simulink subsystem "PWM_BOX"  (R2020b)
settings: Solver=VariableStepAuto  StartTime=0.0  StopTime=10.0  RelTol=1e-3
settings Model: Creator=lee884  LastModifiedBy=lee884

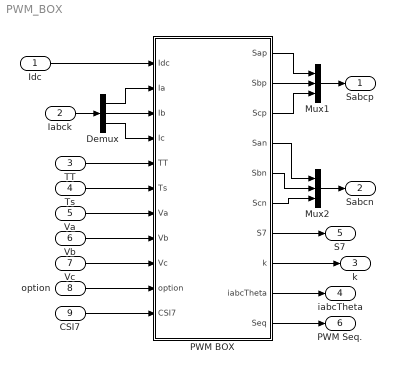
== system PWM_BOX ==
  Idc : Inport
  Iabck : Inport  Port=2
  TT : Inport  Port=3
  Ts : Inport  Port=4
  Va : Inport  Port=5
  Vb : Inport  Port=6
  Vc : Inport  Port=7
  option : Inport  Port=8
  CSI7 : Inport  Port=9
  Demux : Demux  Outputs=3
  Mux1 : Mux  Inputs=3
  Mux2 : Mux  Inputs=3
  PWM BOX : MATLAB Function  TreatAsAtomicUnit=on
  Sabcp : Outport
  Sabcn : Outport  Port=2
  k : Outport  Port=3
  iabcTheta : Outport  Port=4
  S7 : Outport  Port=5
  PWM Seq. : Outport  Port=6
  wires:
  Demux/2 -> PWM BOX/3(Ib)
  PWM BOX/9(iabcTheta) -> iabcTheta/1
  PWM BOX/2(Sbp) -> Mux1/2
  PWM BOX/6(Scn) -> Mux2/3
  PWM BOX/4(San) -> Mux2/1
  Demux/1 -> PWM BOX/2(Ia)
  PWM BOX/5(Sbn) -> Mux2/2
  PWM BOX/3(Scp) -> Mux1/3
  PWM BOX/8(k) -> k/1
  Demux/3 -> PWM BOX/4(Ic)
  TT/1 -> PWM BOX/5(TT)
  PWM BOX/1(Sap) -> Mux1/1
  Mux1/1 -> Sabcp/1
  Ts/1 -> PWM BOX/6(Ts)
  Mux2/1 -> Sabcn/1
  Idc/1 -> PWM BOX/1(Idc)
  Iabck/1 -> Demux/1
  option/1 -> PWM BOX/10(option)
  CSI7/1 -> PWM BOX/11(CSI7)
  PWM BOX/7(S7) -> S7/1
  Va/1 -> PWM BOX/7(Va)
  Vb/1 -> PWM BOX/8(Vb)
  Vc/1 -> PWM BOX/9(Vc)
  PWM BOX/10(Seq) -> PWM Seq./1

== matlab function PWM_BOX/PWM BOX ==
  data: Idc input; Sap output; Sbp output; Scp output; Ia input; Ib input; Ic input; TT input; San output; Ts input; Va input; Vb input; Vc input; Sbn output; Scn output; S7 output; k output; iabcTheta output; option input; CSI7 input; Seq output
function [Sap, Sbp, Scp, San, Sbn, Scn, S7, k,iabcTheta, Seq] = CSI_SVPWM(Idc, Ia, Ib, Ic, TT, Ts, Va, Vb, Vc, option, CSI7)

% S0 = [];
% S1 = [];
% S2 = [];
%% Current space vector
iabc = 2/3 * ( Ia + Ib*exp(1j*2*pi/3) + Ic*exp(1j*4*pi/3) );

%% Sector indentification
iabcTheta = angle (iabc)*180/pi;          % [deg] -180 ~ 180
Seq = 0;
%% CSI switching states
Sab = [1 0 0, 0 1 0];
Sac = [1 0 0, 0 0 1];
Sbc = [0 1 0, 0 0 1];
Sba = [0 1 0, 1 0 0];
Sca = [0 0 1, 1 0 0];
Scb = [0 0 1, 0 1 0];
Saa = [1 0 0, 1 0 0];
Sbb = [0 1 0, 0 1 0];
Scc = [0 0 1, 0 0 1];

%% Sector Identification
k = sector_cal(iabcTheta);

%% Calculate T1, T2, T0 and new T1, T2, T0
[T1, T2, T0] = dwell_time_cal(iabc,iabcTheta,k);
[T1New, T2New] = new_dwell_time_cal(T1, T2, T0);

%% PWM Mapping S0 S1 S2 to switching states
switch option
    case 0
        [Sap, Sbp, Scp, San, Sbn, Scn] = CSM1A(k,TT,Ts,Saa,Sbb,Scc,Sab,Sac,Sbc,Sba,Sca,Scb);
    case 1
        [Sap, Sbp, Scp, San, Sbn, Scn] = DL_CSM1A(k,TT,Ts,Saa,Sbb,Scc,Sab,Sac,Sbc,Sba,Sca,Scb);
    case 2
        [Sap, Sbp, Scp, San, Sbn, Scn] = CSM2A(k,TT,Ts,Saa,Sbb,Scc,Sab,Sac,Sbc,Sba,Sca,Scb);
    case 3
        [Sap, Sbp, Scp, San, Sbn, Scn] = DL_CSM2A(k,TT,Ts,Saa,Sbb,Scc,Sab,Sac,Sbc,Sba,Sca,Scb);
    case 4
        [Sap, Sbp, Scp, San, Sbn, Scn] = CSM3A(k,TT,Ts,Saa,Sbb,Scc,Sab,Sac,Sbc,Sba,Sca,Scb);
        %[Sap, Sbp, Scp, San, Sbn, Scn, S7] = CSM3A_CSI7_with_overlap(k,TT,Ts,Saa,Sbb,Scc,Sab,Sac,Sbc,Sba,Sca,Scb);
    case 5
        [Sap, Sbp, Scp, San, Sbn, Scn] = CSM3A_BoostMinus60deg(k,TT,Ts,Saa,Sbb,Scc,Sab,Sac,Sbc,Sba,Sca,Scb);
    case 6 
        [Sap, Sbp, Scp, San, Sbn, Scn] = AVM(k,TT,Ts,Saa,Sbb,Scc,Sab,Sac,Sbc,Sba,Sca,Scb,Va,Vb,Vc);
    case 7
        [Sap, Sbp, Scp, San, Sbn, Scn] = CSM1B(k,TT,Ts,Saa,Sbb,Scc,Sab,Sac,Sbc,Sba,Sca,Scb);
    case 8
        [Sap, Sbp, Scp, San, Sbn, Scn] = AVM3(k,TT,Ts,Saa,Sbb,Scc,Sab,Sac,Sbc,Sba,Sca,Scb,Va,Vb,Vc);
    otherwise
        [Sap, Sbp, Scp, San, Sbn, Scn, Seq] = ASVM(k,TT,Ts,Saa,Sbb,Scc,Sab,Sac,Sbc,Sba,Sca,Scb,Va,Vb,Vc);        
        
end

%% for CSI7 case, this is the correct modulation of S7 without overlap
if(CSI7 == 1)
    [Sap, Sbp, Scp, San, Sbn, Scn, S7] = S7_modulation(Sap, Sbp, Scp, San, Sbn, Scn);
else
    S7 = 0;
end

% if(option == 4)
%     [Sap, Sbp, Scp, San, Sbn, Scn, S7] = CSM3A_CSI7_with_overlap(k,TT,Ts,Saa,Sbb,Scc,Sab,Sac,Sbc,Sba,Sca,Scb);
% end

%% Define nested functions

    %% Dwell time calculation
    function [T1, T2, T0] = dwell_time_cal(iabc, iabcTheta, k)        
        iabcThetaSector = iabcTheta*pi/180 - (k-1)*pi/3;       % [rad]
        T1 = abs(iabc)/Idc * sin(pi/6-iabcThetaSector) * Ts; 
        T2= abs(iabc)/Idc * sin(pi/6+iabcThetaSector) * Ts; 
        T0 = Ts-T1-T2;
    end

    %% Dwell time calculation for wrong CSI7 or PWAM
    function [T1New, T2New] = new_dwell_time_cal(T1, T2, T0)
        T1New = T1/(T1+T2)*Ts;
        T2New = T2/(T1+T2)*Ts;
    end

    %% Sector number k cacluation
    function k = sector_cal(iabcTheta)
        if iabcTheta > -30 && iabcTheta <= 0; k=1; 
        elseif iabcTheta > 0 && iabcTheta <= 30; k=1;  
    
        % Sector 2
        elseif iabcTheta > 30 && iabcTheta <= 90; k=2; 
    
        % Sector 3
        elseif iabcTheta > 90 && iabcTheta <= 150; k=3; 
    
        % Sector 4
        elseif iabcTheta > 150 && iabcTheta <= 180; k=4; 
        elseif iabcTheta > -180 && iabcTheta <= -150; k=4; 
    
        % Sector 5
        elseif iabcTheta > -150 && iabcTheta <= -90; k=5; 
    
        % Sector 6
        elseif iabcTheta > -90 && iabcTheta <= -30; k=6; 
    
        % Else- Error
        else k = 10; 
        end        
    end



%%%%%%%%%%%%%%%%%%%%%%%%%%%%%%%%%%%%%%%%%%%%%%%%% PWM logics
%%%%%%%%%%%%%%%%%%%%%%%%%%%%%%%%%%%%%%%%%%%%%%%%% %%%%%%%%%%%%%%%%%%%%%%%%%%%%%%%%%%%%%%%
%% CSM1A: IZ-IA-IB-IA-IZ
% CSM1A
    function [Sap, Sbp, Scp, San, Sbn, Scn] = CSM1A(k,TT,Ts,Saa,Sbb,Scc,Sab,Sac,Sbc,Sba,Sca,Scb)
        
        switch k
            case 1
                S0 = Saa; S1 = Sab; S2 = Sac;
            case 2
                S0 = Scc; S1 = Sac; S2 = Sbc;
            case 3
                S0 = Sbb; S1 = Sbc; S2 = Sba;
            case 4
                S0 = Saa; S1 = Sba; S2 = Sca;
            case 5
                S0 = Scc; S1 = Sca; S2 = Scb;
            case 6
                S0 = Sbb; S1 = Scb; S2 = Sab;
            otherwise
                S0 = Saa; S1 = Sab; S2 = Sac;
        end
        
        
        % initialize switching functions
        Sap = 1; Sbp = 1; Scp = 1;
        San = 1; Sbn = 1; Scn = 1;
        
        % PWM sequence: IZ-IA-IB-IA-IZ
        if TT>=0 && TT<T0/2
            % aa or bb or cc, CSI zero state
            Sap = S0(1);    Sbp = S0(2);    Scp = S0(3);
            San = S0(4);    Sbn = S0(5);    Scn = S0(6);

        elseif TT>=T0/2 && TT<T0/2 + T1/2
            % T1 state
            Sap = S1(1);    Sbp = S1(2);    Scp = S1(3);
            San = S1(4);    Sbn = S1(5);    Scn = S1(6);    

        elseif TT>=T0/2 + T1/2 && TT<=T0/2 + T1/2 +T2 
            % T2 state
            Sap = S2(1);    Sbp = S2(2);    Scp = S2(3);
            San = S2(4);    Sbn = S2(5);    Scn = S2(6);
    
        elseif TT>=T0/2 + T1/2 +T2 && TT<T0/2 + T1 +T2
            % T1 state
            Sap = S1(1);    Sbp = S1(2);    Scp = S1(3);
            San = S1(4);    Sbn = S1(5);    Scn = S1(6);

        elseif TT>=T0/2 + T1 +T2 && TT<Ts
            % aa or bb or cc, CSI zero state
            Sap = S0(1);    Sbp = S0(2);    Scp = S0(3);
            San = S0(4);    Sbn = S0(5);    Scn = S0(6);
        end        
    end

%% CSM1B: IZ-IB-IA-IB-IZ
% CSM1B
    function [Sap, Sbp, Scp, San, Sbn, Scn] = CSM1B(k,TT,Ts,Saa,Sbb,Scc,Sab,Sac,Sbc,Sba,Sca,Scb)
        
        switch k
            case 1
                S0 = Saa; S1 = Sab; S2 = Sac;
            case 2
                S0 = Scc; S1 = Sac; S2 = Sbc;
            case 3
                S0 = Sbb; S1 = Sbc; S2 = Sba;
            case 4
                S0 = Saa; S1 = Sba; S2 = Sca;
            case 5
                S0 = Scc; S1 = Sca; S2 = Scb;
            case 6
                S0 = Sbb; S1 = Scb; S2 = Sab;
            otherwise
                S0 = Saa; S1 = Sab; S2 = Sac;
        end
        
        
        % initialize switching functions
        Sap = 1; Sbp = 1; Scp = 1;
        San = 1; Sbn = 1; Scn = 1;
        
        % PWM sequence: IZ-IB-IA-IB-IZ
        if TT>=0 && TT<T0/2
            % aa or bb or cc, CSI zero state
            Sap = S0(1);    Sbp = S0(2);    Scp = S0(3);
            San = S0(4);    Sbn = S0(5);    Scn = S0(6);

        elseif TT>=T0/2 && TT<T0/2 + T2/2
            % T1 state
            Sap = S2(1);    Sbp = S2(2);    Scp = S2(3);
            San = S2(4);    Sbn = S2(5);    Scn = S2(6);    

        elseif TT>=T0/2 + T2/2 && TT<=T0/2 + T2/2 +T1 
            % T2 state
            Sap = S1(1);    Sbp = S1(2);    Scp = S1(3);
            San = S1(4);    Sbn = S1(5);    Scn = S1(6);
    
        elseif TT>=T0/2 + T2/2 +T1 && TT<T0/2 + T2 +T1
            % T1 state
            Sap = S2(1);    Sbp = S2(2);    Scp = S2(3);
            San = S2(4);    Sbn = S2(5);    Scn = S2(6);

        elseif TT>=T0/2 + T2 + T1 && TT<Ts
            % aa or bb or cc, CSI zero state
            Sap = S0(1);    Sbp = S0(2);    Scp = S0(3);
            San = S0(4);    Sbn = S0(5);    Scn = S0(6);
        end        
    end

%% DL-CSM1A: IZ-IA-IB-IA-IZ
% DL-CSM1A
    function [Sap, Sbp, Scp, San, Sbn, Scn] = DL_CSM1A(k,TT,Ts,Saa,Sbb,Scc,Sab,Sac,Sbc,Sba,Sca,Scb)
        switch k
            case 1
                S0 = Sbb; S1 = Sab; S2 = Sac;
            case 2
                S0 = Saa; S1 = Sac; S2 = Sbc;
            case 3
                S0 = Scc; S1 = Sbc; S2 = Sba;
            case 4
                S0 = Sbb; S1 = Sba; S2 = Sca;
            case 5
                S0 = Saa; S1 = Sca; S2 = Scb;
            case 6
                S0 = Scc; S1 = Scb; S2 = Sab;
            otherwise
                S0 = Saa; S1 = Sab; S2 = Sac;
        end

        % initialize switching functions
        Sap = 1; Sbp = 1; Scp = 1;
        San = 1; Sbn = 1; Scn = 1;        
        
        % PWM sequence: IZ-IA-IB-IA-IZ
        if TT>=0 && TT<T0/2
            % aa or bb or cc, CSI zero state
            Sap = S0(1);    Sbp = S0(2);    Scp = S0(3);
            San = S0(4);    Sbn = S0(5);    Scn = S0(6);

        elseif TT>=T0/2 && TT<T0/2 + T1/2
            % T1 state
            Sap = S1(1);    Sbp = S1(2);    Scp = S1(3);
            San = S1(4);    Sbn = S1(5);    Scn = S1(6);    

        elseif TT>=T0/2 + T1/2 && TT<=T0/2 + T1/2 +T2 
            % T2 state
            Sap = S2(1);    Sbp = S2(2);    Scp = S2(3);
            San = S2(4);    Sbn = S2(5);    Scn = S2(6);
    
        elseif TT>=T0/2 + T1/2 +T2 && TT<T0/2 + T1 +T2
            % T1 state
            Sap = S1(1);    Sbp = S1(2);    Scp = S1(3);
            San = S1(4);    Sbn = S1(5);    Scn = S1(6);

        elseif TT>=T0/2 + T1 +T2 && TT<Ts
            % aa or bb or cc, CSI zero state
            Sap = S0(1);    Sbp = S0(2);    Scp = S0(3);
            San = S0(4);    Sbn = S0(5);    Scn = S0(6);
        end  
    end

%% CSM2A: IA-IB-IZ-IB-IA
% CSM1A
    function [Sap, Sbp, Scp, San, Sbn, Scn] = CSM2A(k,TT,Ts,Saa,Sbb,Scc,Sab,Sac,Sbc,Sba,Sca,Scb)
        

        switch k
            case 1
                S0 = Saa; S1 = Sab; S2 = Sac;
            case 2
                S0 = Scc; S1 = Sac; S2 = Sbc;
            case 3
                S0 = Sbb; S1 = Sbc; S2 = Sba;
            case 4
                S0 = Saa; S1 = Sba; S2 = Sca;
            case 5
                S0 = Scc; S1 = Sca; S2 = Scb;
            case 6
                S0 = Sbb; S1 = Scb; S2 = Sab;
            otherwise
                S0 = Saa; S1 = Sab; S2 = Sac;
        end
        
        
        % initialize switching functions
        Sap = 1; Sbp = 1; Scp = 1;
        San = 1; Sbn = 1; Scn = 1;
        
        % PWM sequence: IA-IB-IZ-IB-IA
        if TT>=0 && TT<T1/2
            % aa or bb or cc, CSI zero state
            Sap = S1(1);    Sbp = S1(2);    Scp = S1(3);
            San = S1(4);    Sbn = S1(5);    Scn = S1(6);

        elseif TT>=T1/2 && TT<T1/2 + T2/2
            % T1 state
            Sap = S2(1);    Sbp = S2(2);    Scp = S2(3);
            San = S2(4);    Sbn = S2(5);    Scn = S2(6);    

        elseif TT>=T1/2 + T2/2 && TT<=T1/2 + T2/2 + T0 
            % T2 state
            Sap = S0(1);    Sbp = S0(2);    Scp = S0(3);
            San = S0(4);    Sbn = S0(5);    Scn = S0(6);
    
        elseif TT>=T1/2 + T2/2 + T0 && TT<T1/2 + T2 +T0
            % T1 state
            Sap = S2(1);    Sbp = S2(2);    Scp = S2(3);
            San = S2(4);    Sbn = S2(5);    Scn = S2(6);

        elseif TT>=T1/2 + T2 +T0 && TT<Ts
            % aa or bb or cc, CSI zero state
            Sap = S1(1);    Sbp = S1(2);    Scp = S1(3);
            San = S1(4);    Sbn = S1(5);    Scn = S1(6);
        end        
    end

%% DL-CSM2A: IA-IB-IZ-IB-IA
% DL-CSM2A
    function [Sap, Sbp, Scp, San, Sbn, Scn] = DL_CSM2A(k,TT,Ts,Saa,Sbb,Scc,Sab,Sac,Sbc,Sba,Sca,Scb)
        switch k
            case 1
                S0 = Scc; S1 = Sab; S2 = Sac;
            case 2
                S0 = Sbb; S1 = Sac; S2 = Sbc;
            case 3
                S0 = Saa; S1 = Sbc; S2 = Sba;
            case 4
                S0 = Scc; S1 = Sba; S2 = Sca;
            case 5
                S0 = Sbb; S1 = Sca; S2 = Scb;
            case 6
                S0 = Saa; S1 = Scb; S2 = Sab;
            otherwise
                S0 = Saa; S1 = Sab; S2 = Sac;
        end

        % initialize switching functions
        Sap = 1; Sbp = 1; Scp = 1;
        San = 1; Sbn = 1; Scn = 1;        
        
        % PWM sequence: IA-IB-IZ-IB-IA
        if TT>=0 && TT<T1/2
            % aa or bb or cc, CSI zero state
            Sap = S1(1);    Sbp = S1(2);    Scp = S1(3);
            San = S1(4);    Sbn = S1(5);    Scn = S1(6);

        elseif TT>=T1/2 && TT<T1/2 + T2/2
            % T1 state
            Sap = S2(1);    Sbp = S2(2);    Scp = S2(3);
            San = S2(4);    Sbn = S2(5);    Scn = S2(6);    

        elseif TT>=T1/2 + T2/2 && TT<=T1/2 + T2/2 +T0 
            % T2 state
            Sap = S0(1);    Sbp = S0(2);    Scp = S0(3);
            San = S0(4);    Sbn = S0(5);    Scn = S0(6);
    
        elseif TT>=T1/2 + T2/2 +T0 && TT<T1/2 + T2 +T0
            % T1 state
            Sap = S2(1);    Sbp = S2(2);    Scp = S2(3);
            San = S2(4);    Sbn = S2(5);    Scn = S2(6);

        elseif TT>=T1/2 + T2 +T0 && TT<Ts
            % aa or bb or cc, CSI zero state
            Sap = S1(1);    Sbp = S1(2);    Scp = S1(3);
            San = S1(4);    Sbn = S1(5);    Scn = S1(6);
        end  
    end

%% CSI7 or PWAM: IZ-IA-IB-IA-IZ
% Wrong CSI7 modulation
    function [Sap, Sbp, Scp, San, Sbn, Scn, S7] = CSM3A_CSI7_with_overlap(k,TT,Ts,Saa,Sbb,Scc,Sab,Sac,Sbc,Sba,Sca,Scb)
        
        switch k
            case 1
                S0 = Saa; S1 = Sab; S2 = Sac;
            case 2
                S0 = Scc; S1 = Sac; S2 = Sbc;
            case 3
                S0 = Sbb; S1 = Sbc; S2 = Sba;
            case 4
                S0 = Saa; S1 = Sba; S2 = Sca;
            case 5
                S0 = Scc; S1 = Sca; S2 = Scb;
            case 6
                S0 = Sbb; S1 = Scb; S2 = Sab;
            otherwise
                S0 = Saa; S1 = Sab; S2 = Sac;
        end

        % initialize switching functions
        Sap = 1; Sbp = 1; Scp = 1;
        San = 1; Sbn = 1; Scn = 1; 
        S7 = 0;

        % PWM sequence for CSI switch : IZ-IA-IB-IA-IZ
        if TT>=0 && TT<T1New/2
            % aa or bb or cc, CSI zero state
            Sap = S1(1);    Sbp = S1(2);    Scp = S1(3);
            San = S1(4);    Sbn = S1(5);    Scn = S1(6);

        elseif TT>=T1New/2 && TT<T1New/2 + T2New
            % T1 state
            Sap = S2(1);    Sbp = S2(2);    Scp = S2(3);
            San = S2(4);    Sbn = S2(5);    Scn = S2(6);

        elseif TT>=T1New/2 + T2New && TT<Ts 
            % T2 state
            Sap = S1(1);    Sbp = S1(2);    Scp = S1(3);
            San = S1(4);    Sbn = S1(5);    Scn = S1(6);
        end           
        
        
        % PWM sequence for S7 : IZ-IA-IB-IA-IZ
        if TT>=0 && TT<T1/2
            % T1 state
            S7 = 0;

        elseif TT>=T1/2 && TT<T1/2 + T0/2
            % aa or bb or cc, CSI zero state
            S7 = 1;

        elseif TT>=T1/2 + T0/2 && TT< T1/2 + T0/2 +T2 
            % T2 state
            S7 = 0;
    
        elseif TT>=T1/2 + T0/2 +T2 && TT<T1/2 + T0 +T2
            % aa or bb or cc, CSI zero state
            S7 = 1;

        elseif TT>=T1/2 + T0 +T2 && TT<Ts
            % T1 state  
            S7 = 0;
        end        
    end

%% CSM3A IA-IZ-IB-IZ-IA
% CSM3
    function [Sap, Sbp, Scp, San, Sbn, Scn] = CSM3A(k,TT,Ts,Saa,Sbb,Scc,Sab,Sac,Sbc,Sba,Sca,Scb)

        switch k
            case 1
                S0 = Saa; S1 = Sab; S2 = Sac;
            case 2
                S0 = Scc; S1 = Sac; S2 = Sbc;
            case 3
                S0 = Sbb; S1 = Sbc; S2 = Sba;
            case 4
                S0 = Saa; S1 = Sba; S2 = Sca;
            case 5
                S0 = Scc; S1 = Sca; S2 = Scb;
            case 6
                S0 = Sbb; S1 = Scb; S2 = Sab;
            otherwise
                S0 = Saa; S1 = Sab; S2 = Sac;
        end
        
        
        % initialize switching functions
        Sap = 1; Sbp = 1; Scp = 1;
        San = 1; Sbn = 1; Scn = 1;
        
        % PWM sequence: IA-IZ-IB-IZ-IA
        if TT>=0 && TT<T1/2
            % T1
            Sap = S1(1);    Sbp = S1(2);    Scp = S1(3);
            San = S1(4);    Sbn = S1(5);    Scn = S1(6);

        elseif TT>=T1/2 && TT<T1/2 + T0/2
            % T0
            Sap = S0(1);    Sbp = S0(2);    Scp = S0(3);
            San = S0(4);    Sbn = S0(5);    Scn = S0(6);    

        elseif TT>=T1/2 + T2/2 && TT<=T1/2 + T0/2 + T2 
            % T2
            Sap = S2(1);    Sbp = S2(2);    Scp = S2(3);
            San = S2(4);    Sbn = S2(5);    Scn = S2(6);
    
        elseif TT>=T1/2 + T0/2 + T2 && TT<T1/2 + T2 +T0
            % T0
            Sap = S0(1);    Sbp = S0(2);    Scp = S0(3);
            San = S0(4);    Sbn = S0(5);    Scn = S0(6);

        elseif TT>=T1/2 + T2 +T0 && TT<Ts
            % T1
            Sap = S1(1);    Sbp = S1(2);    Scp = S1(3);
            San = S1(4);    Sbn = S1(5);    Scn = S1(6);
        end        
    end

%% S7 modulation with direct replacment of zero vectors
    function [Sap, Sbp, Scp, San, Sbn, Scn, S7] = S7_modulation(Sap, Sbp, Scp, San, Sbn, Scn)
         S7 = 0;
         if(Sap == 1 && San ==1)
             S7 = 1;
             Sap = 0; San = 0;
         end
         
         if(Sbp == 1 && Sbn ==1)
             S7 = 1;
             Sbp = 0; Sbn = 0;
         end
         
         if(Scp == 1 && Scn ==1)
             S7 = 1;
             Scp = 0; Scn = 0;
         end
         
    end

%% boost operation modulation CSM3A IA-IZ-IB-IZ-IA with negative
    function [Sap, Sbp, Scp, San, Sbn, Scn] = CSM3A_BoostMinus60deg(k,TT,Ts,Saa,Sbb,Scc,Sab,Sac,Sbc,Sba,Sca,Scb)
        
        switch k
            case 1
                S0 = Saa; S1 = Sab; S2 = Sbc;
            case 2
                S0 = Scc; S1 = Sac; S2 = Sba;
            case 3
                S0 = Sbb; S1 = Sbc; S2 = Sca;
            case 4
                S0 = Saa; S1 = Sba; S2 = Scb;
            case 5
                S0 = Scc; S1 = Sca; S2 = Sab;
            case 6
                S0 = Sbb; S1 = Scb; S2 = Sac;
            otherwise
                S0 = Saa; S1 = Sab; S2 = Sac;
        end

        % initialize switching functions
        Sap = 1; Sbp = 1; Scp = 1;
        San = 1; Sbn = 1; Scn = 1; 
        S7 = 0;
        
        % For 60 deg T1 becomes T1 + T2 and T2 becomes T2
        T1new = T1 + T2;
        T2new = T2;
        T0new = Ts - T1new - T2new;
        
        % PWM sequence for CSI switch : IA-IZ-IB-IZ-IA
        if TT>=0 && TT<T1new/2
            % T1 state
            Sap = S1(1);    Sbp = S1(2);    Scp = S1(3);
            San = S1(4);    Sbn = S1(5);    Scn = S1(6);

        elseif TT>=T1new/2 && TT<T1new/2 + T0new/2
            % T0 state
            Sap = S0(1);    Sbp = S0(2);    Scp = S0(3);
            San = S0(4);    Sbn = S0(5);    Scn = S0(6);

        elseif TT>=T1new/2 + T0new/2 && TT<T1new/2 + T0new/2 + T2new 
            % T2 state
            Sap = S2(1);    Sbp = S2(2);    Scp = S2(3);
            San = S2(4);    Sbn = S2(5);    Scn = S2(6);
            
        elseif TT>=T1new/2 + T0new/2 + T2new && TT<T1new/2 + T0new + T2new
            % T0 state
            Sap = S0(1);    Sbp = S0(2);    Scp = S0(3);
            San = S0(4);    Sbn = S0(5);    Scn = S0(6);
            
        elseif TT>=T1new/2 + T0new + T2new && TT<Ts
            % T1 state
            Sap = S1(1);    Sbp = S1(2);    Scp = S1(3);
            San = S1(4);    Sbn = S1(5);    Scn = S1(6);
        end         
    end

%% boost operation modulation CSM3A IA-IZ-IB-IZ-IA with positive
    function [Sap, Sbp, Scp, San, Sbn, Scn] = CSM3A_BoostPositive60deg(k,TT,Ts,Saa,Sbb,Scc,Sab,Sac,Sbc,Sba,Sca,Scb)
        
        switch k
            case 1
                S0 = Saa; S1 = Scb; S2 = Sac;
            case 2
                S0 = Scc; S1 = Sab; S2 = Sbc;
            case 3
                S0 = Sbb; S1 = Sac; S2 = Sba;
            case 4
                S0 = Saa; S1 = Sbc; S2 = Sca;
            case 5
                S0 = Scc; S1 = Sba; S2 = Scb;
            case 6
                S0 = Sbb; S1 = Sca; S2 = Sab;
            otherwise
                S0 = Saa; S1 = Scb; S2 = Sac;
        end

        % initialize switching functions
        Sap = 1; Sbp = 1; Scp = 1;
        San = 1; Sbn = 1; Scn = 1; 
        S7 = 0;
        
        % For 60 deg T1 becomes T1 + T2 and T2 becomes T2
        T1new = T1;
        T2new = T1 + T2;
        T0new = Ts - T1new - T2new;
        
        % PWM sequence for CSI switch : IA-IZ-IB-IZ-IA
        if TT>=0 && TT<T1new/2
            % T1 state
            Sap = S1(1);    Sbp = S1(2);    Scp = S1(3);
            San = S1(4);    Sbn = S1(5);    Scn = S1(6);

        elseif TT>=T1new/2 && TT<T1new/2 + T0new/2
            % T0 state
            Sap = S0(1);    Sbp = S0(2);    Scp = S0(3);
            San = S0(4);    Sbn = S0(5);    Scn = S0(6);

        elseif TT>=T1new/2 + T0new/2 && TT<T1new/2 + T0new/2 + T2new 
            % T2 state
            Sap = S2(1);    Sbp = S2(2);    Scp = S2(3);
            San = S2(4);    Sbn = S2(5);    Scn = S2(6);
            
        elseif TT>=T1new/2 + T0new/2 + T2new && TT<T1new/2 + T0new + T2new
            % T0 state
            Sap = S0(1);    Sbp = S0(2);    Scp = S0(3);
            San = S0(4);    Sbn = S0(5);    Scn = S0(6);
            
        elseif TT>=T1new/2 + T0new + T2new && TT<Ts
            % T1 state
            Sap = S1(1);    Sbp = S1(2);    Scp = S1(3);
            San = S1(4);    Sbn = S1(5);    Scn = S1(6);
        end         
    end

%% AVM: IZ-IA-IB-IA-IZ (2023 ECCE)
% AVM
    function [Sap, Sbp, Scp, San, Sbn, Scn] = AVM(k,TT,Ts,Saa,Sbb,Scc,Sab,Sac,Sbc,Sba,Sca,Scb,Va,Vb,Vc)
        Va_mag = abs(Va);
        Vb_mag = abs(Vb);
        Vc_mag = abs(Vc);
        
        if(Va_mag >= Vb_mag && Vb_mag >= Vc_mag)
            n = 1; m = 1; % |Va| >= |Vb| >= |Vc|
        elseif(Va_mag >= Vc_mag && Vc_mag >= Vb_mag)
            n = 2; m = 1; % |Va| >= |Vc| > |Vb|
        elseif(Vb_mag >= Va_mag && Va_mag >= Vc_mag)
            n = 3; m = 2; % |Vb| >= |Va| > |Vc|
        elseif(Vb_mag >= Vc_mag && Vc_mag >= Va_mag)
            n = 4; m = 2; % |Vb| > |Vc| > |Va|
        elseif(Vc_mag >= Va_mag && Va_mag >= Vb_mag)
            n = 5; m = 3; % |Vc| > |Va| > |Vb|
        else            
            n = 6; m = 3; % |Vc| > |Vb| > |Va|
        end
        
%% Select the right active vectors       
        switch k
            case 1 % Sector I
                switch m
                    case 1 % |Va| is max
                        S0 = Saa; S1 = Sab; S2 = Sac; SQ = 2;
                    case 2 % |Vb| is max
                        S0 = Saa; S1 = Sab; S2 = Sbc; SQ = 3;
                    otherwise % |Vc| is max
                        S0 = Saa; S1 = Scb; S2 = Sac; SQ = 1;
                end                
            case 2
                switch m
                    case 1 % |Va| is max
                        S0 = Scc; S1 = Sac; S2 = Sba; SQ = 3;
                    case 2 % |Vb| is max
                        S0 = Scc; S1 = Sab; S2 = Sbc; SQ = 1;
                    otherwise % |Vc| is max
                        S0 = Scc; S1 = Sac; S2 = Sbc; SQ = 2;
                end    
            case 3
                switch m
                    case 1 % |Va| is max
                        S0 = Sbb; S1 = Sac; S2 = Sba; SQ = 1;
                    case 2 % |Vb| is max
                        S0 = Sbb; S1 = Sbc; S2 = Sba; SQ = 2;
                    otherwise % |Vc| is max
                        S0 = Sbb; S1 = Sbc; S2 = Sca; SQ = 3;
                end
            case 4
                switch m
                    case 1 % |Va| is max
                        S0 = Saa; S1 = Sba; S2 = Sca; SQ = 2;
                    case 2 % |Vb| is max
                        S0 = Saa; S1 = Sba; S2 = Scb; SQ = 3;
                    otherwise % |Vc| is max
                        S0 = Saa; S1 = Sbc; S2 = Sca; SQ = 1;
                end
            case 5
                switch m
                    case 1 % |Va| is max
                        S0 = Scc; S1 = Sca; S2 = Sab; SQ = 3;
                    case 2 % |Vb| is max
                        S0 = Scc; S1 = Sba; S2 = Scb; SQ = 1;
                    otherwise % |Vc| is max
                        S0 = Scc; S1 = Sca; S2 = Scb; SQ = 2;
                end
            case 6
                switch m
                    case 1 % |Va| is max
                        S0 = Sbb; S1 = Sca; S2 = Sab; SQ = 1;
                    case 2 % |Vb| is max
                        S0 = Sbb; S1 = Scb; S2 = Sab; SQ = 2;
                    otherwise % |Vc| is max
                        S0 = Sbb; S1 = Scb; S2 = Sac; SQ = 3;
                end               
            otherwise
                S0 = Saa; S1 = Sab; S2 = Sac; SQ = 0
        end
        
%%        
        % initialize switching functions
        Sap = 1; Sbp = 1; Scp = 1;
        San = 1; Sbn = 1; Scn = 1;

        % Calculate T1 T2 for SQ1 and SQ3
        T1_SQ1 = T1;
        T2_SQ1 = T1 + T2;
        T0_SQ1 = Ts - T1_SQ1 - T2_SQ1;
        
        T1_SQ3 = T1 + T2;
        T2_SQ3 = T2;
        T0_SQ3 = Ts - T1_SQ3 - T2_SQ3;
        
        % Assign TZ TA TB
        switch SQ
            case 1
                TZ = T0_SQ1; TA = T1_SQ1; TB = T2_SQ1;
            case 2
                TZ = T0; TA = T1; TB = T2;
            otherwise
                TZ = T0_SQ3; TA = T1_SQ3; TB = T2_SQ3;                
        end
        
        % PWM sequence
        if(SQ == 1) % PWM sequence: IZ-IB-IA-IB-IZ
            if TT>=0 && TT<TZ/2
                % aa or bb or cc, CSI zero state
                Sap = S0(1);    Sbp = S0(2);    Scp = S0(3);
                San = S0(4);    Sbn = S0(5);    Scn = S0(6);

            elseif TT>=TZ/2 && TT<TZ/2 + TB/2
                % T2 state
                Sap = S2(1);    Sbp = S2(2);    Scp = S2(3);
                San = S2(4);    Sbn = S2(5);    Scn = S2(6);    

            elseif TT>=TZ/2 + TB/2 && TT<=TZ/2 + TB/2 + TA 
                % T1 state
                Sap = S1(1);    Sbp = S1(2);    Scp = S1(3);
                San = S1(4);    Sbn = S1(5);    Scn = S1(6);
    
            elseif TT>=TZ/2 + TB/2 + TA && TT<TZ/2 + TA + TB
                % T2 state
                Sap = S2(1);    Sbp = S2(2);    Scp = S2(3);
                San = S2(4);    Sbn = S2(5);    Scn = S2(6);

            elseif TT>=TZ/2 + TA + TB && TT<Ts
                % aa or bb or cc, CSI zero state
                Sap = S0(1);    Sbp = S0(2);    Scp = S0(3);
                San = S0(4);    Sbn = S0(5);    Scn = S0(6);
            end 
        else % SQ2 and SQ3      
            % PWM sequence: IZ-IA-IB-IA-IZ
            if TT>=0 && TT<TZ/2
                % aa or bb or cc, CSI zero state
                Sap = S0(1);    Sbp = S0(2);    Scp = S0(3);
                San = S0(4);    Sbn = S0(5);    Scn = S0(6);

            elseif TT>=TZ/2 && TT<TZ/2 + TA/2
                % T1 state
                Sap = S1(1);    Sbp = S1(2);    Scp = S1(3);
                San = S1(4);    Sbn = S1(5);    Scn = S1(6);    

            elseif TT>=TZ/2 + TA/2 && TT<=TZ/2 + TA/2 + TB 
                % T2 state
                Sap = S2(1);    Sbp = S2(2);    Scp = S2(3);
                San = S2(4);    Sbn = S2(5);    Scn = S2(6);
    
            elseif TT>=TZ/2 + TA/2 + TB && TT<TZ/2 + TA +TB
                % T1 state
                Sap = S1(1);    Sbp = S1(2);    Scp = S1(3);
                San = S1(4);    Sbn = S1(5);    Scn = S1(6);

            elseif TT>=TZ/2 + TA + TB && TT<Ts
                % aa or bb or cc, CSI zero state
                Sap = S0(1);    Sbp = S0(2);    Scp = S0(3);
                San = S0(4);    Sbn = S0(5);    Scn = S0(6);
            end 
        end
        
        
    end

%% AVM3: IA-IZ-IB-IZ-IA (2023 ECCE converting to Journal with CSI7)
% AVM3
    function [Sap, Sbp, Scp, San, Sbn, Scn] = AVM3(k,TT,Ts,Saa,Sbb,Scc,Sab,Sac,Sbc,Sba,Sca,Scb,Va,Vb,Vc)
        Va_mag = abs(Va);
        Vb_mag = abs(Vb);
        Vc_mag = abs(Vc);
        
        if(Va_mag >= Vb_mag && Vb_mag >= Vc_mag)
            n = 1; m = 1; % |Va| >= |Vb| >= |Vc|
        elseif(Va_mag >= Vc_mag && Vc_mag >= Vb_mag)
            n = 2; m = 1; % |Va| >= |Vc| > |Vb|
        elseif(Vb_mag >= Va_mag && Va_mag >= Vc_mag)
            n = 3; m = 2; % |Vb| >= |Va| > |Vc|
        elseif(Vb_mag >= Vc_mag && Vc_mag >= Va_mag)
            n = 4; m = 2; % |Vb| > |Vc| > |Va|
        elseif(Vc_mag >= Va_mag && Va_mag >= Vb_mag)
            n = 5; m = 3; % |Vc| > |Va| > |Vb|
        else            
            n = 6; m = 3; % |Vc| > |Vb| > |Va|
        end
        
%% Select the right active vectors       
        switch k
            case 1 % Sector I
                switch m
                    case 1 % |Va| is max
                        S0 = Saa; S1 = Sab; S2 = Sac; SQ = 2;
                    case 2 % |Vb| is max
                        S0 = Saa; S1 = Sab; S2 = Sbc; SQ = 3;
                    otherwise % |Vc| is max
                        S0 = Saa; S1 = Scb; S2 = Sac; SQ = 1;
                end                
            case 2
                switch m
                    case 1 % |Va| is max
                        S0 = Scc; S1 = Sac; S2 = Sba; SQ = 3;
                    case 2 % |Vb| is max
                        S0 = Scc; S1 = Sab; S2 = Sbc; SQ = 1;
                    otherwise % |Vc| is max
                        S0 = Scc; S1 = Sac; S2 = Sbc; SQ = 2;
                end    
            case 3
                switch m
                    case 1 % |Va| is max
                        S0 = Sbb; S1 = Sac; S2 = Sba; SQ = 1;
                    case 2 % |Vb| is max
                        S0 = Sbb; S1 = Sbc; S2 = Sba; SQ = 2;
                    otherwise % |Vc| is max
                        S0 = Sbb; S1 = Sbc; S2 = Sca; SQ = 3;
                end
            case 4
                switch m
                    case 1 % |Va| is max
                        S0 = Saa; S1 = Sba; S2 = Sca; SQ = 2;
                    case 2 % |Vb| is max
                        S0 = Saa; S1 = Sba; S2 = Scb; SQ = 3;
                    otherwise % |Vc| is max
                        S0 = Saa; S1 = Sbc; S2 = Sca; SQ = 1;
                end
            case 5
                switch m
                    case 1 % |Va| is max
                        S0 = Scc; S1 = Sca; S2 = Sab; SQ = 3;
                    case 2 % |Vb| is max
                        S0 = Scc; S1 = Sba; S2 = Scb; SQ = 1;
                    otherwise % |Vc| is max
                        S0 = Scc; S1 = Sca; S2 = Scb; SQ = 2;
                end
            case 6
                switch m
                    case 1 % |Va| is max
                        S0 = Sbb; S1 = Sca; S2 = Sab; SQ = 1;
                    case 2 % |Vb| is max
                        S0 = Sbb; S1 = Scb; S2 = Sab; SQ = 2;
                    otherwise % |Vc| is max
                        S0 = Sbb; S1 = Scb; S2 = Sac; SQ = 3;
                end               
            otherwise
                S0 = Saa; S1 = Sab; S2 = Sac; SQ = 0;
        end
        
%%        
        % initialize switching functions
        Sap = 1; Sbp = 1; Scp = 1;
        San = 1; Sbn = 1; Scn = 1;

        % Calculate T1 T2 for SQ1 and SQ3
        T1_SQ1 = T1;
        T2_SQ1 = T1 + T2;
        T0_SQ1 = Ts - T1_SQ1 - T2_SQ1;
        
        T1_SQ3 = T1 + T2;
        T2_SQ3 = T2;
        T0_SQ3 = Ts - T1_SQ3 - T2_SQ3;
        
        % Assign TZ TA TB
        switch SQ
            case 1
                TZ = T0_SQ1; TA = T1_SQ1; TB = T2_SQ1;
            case 2
                TZ = T0; TA = T1; TB = T2;
            otherwise
                TZ = T0_SQ3; TA = T1_SQ3; TB = T2_SQ3;                
        end
        
        % PWM sequence: IA-IZ-IB-IZ-IA
            if TT>=0 && TT<TA/2
                % T1
                Sap = S1(1);    Sbp = S1(2);    Scp = S1(3);
                San = S1(4);    Sbn = S1(5);    Scn = S1(6);

            elseif TT>=TA/2 && TT<TA/2 + TZ/2
                % T0
                Sap = S0(1);    Sbp = S0(2);    Scp = S0(3);
                San = S0(4);    Sbn = S0(5);    Scn = S0(6);    

            elseif TT>=TA/2 + TZ/2 && TT<=TA/2 + TZ/2 + TB 
                % T2
                Sap = S2(1);    Sbp = S2(2);    Scp = S2(3);
                San = S2(4);    Sbn = S2(5);    Scn = S2(6);
    
            elseif TT>=TA/2 + TZ/2 + TB && TT<TA/2 + TZ + TB
                % T0 state
                Sap = S0(1);    Sbp = S0(2);    Scp = S0(3);
                San = S0(4);    Sbn = S0(5);    Scn = S0(6);

            elseif TT>=TA/2 + TZ + TB && TT<Ts
                % T1
                Sap = S1(1);    Sbp = S1(2);    Scp = S1(3);
                San = S1(4);    Sbn = S1(5);    Scn = S1(6);
            end        
    end

%% AVZM3: AVM with improved zero current vector: IA-IZ-IB-IZ-IA (2023 ECCE converting to Journal with CSI7)
% AVZM3
    function [Sap, Sbp, Scp, San, Sbn, Scn] = AVZM3(k,TT,Ts,Saa,Sbb,Scc,Sab,Sac,Sbc,Sba,Sca,Scb,Va,Vb,Vc)
        Va_mag = abs(Va);
        Vb_mag = abs(Vb);
        Vc_mag = abs(Vc);
        
        if(Va_mag >= Vb_mag && Vb_mag >= Vc_mag)
            % |Va| >= |Vb| >= |Vc|
            n = 3; 
            m = 1; % |Va| is max
        elseif(Va_mag >= Vc_mag && Vc_mag >= Vb_mag)
            % |Va| >= |Vc| > |Vb|
            n = 2; 
            m = 1; % |Va| is max 
        elseif(Vb_mag >= Va_mag && Va_mag >= Vc_mag)
             % |Vb| >= |Va| > |Vc|
            n = 3; 
            m = 2; % |Vb| is max
        elseif(Vb_mag >= Vc_mag && Vc_mag >= Va_mag)
            % |Vb| > |Vc| > |Va|
            n = 1; 
            m = 2; % |Vb| is max
        elseif(Vc_mag >= Va_mag && Va_mag >= Vb_mag)
            % |Vc| > |Va| > |Vb|
            n = 2; 
            m = 3; % |Vc| is max
        else          
            % |Vc| > |Vb| > |Va|
            n = 1; 
            m = 3; % |Vc| is max
        end
        
%% Select the right active vectors       
        switch k
            case 1 % Sector I
                switch m
                    case 1 % |Va| is max
                        S0 = Saa; S1 = Sab; S2 = Sac; SQ = 2;
                    case 2 % |Vb| is max
                        S0 = Saa; S1 = Sab; S2 = Sbc; SQ = 3;
                    otherwise % |Vc| is max
                        S0 = Saa; S1 = Scb; S2 = Sac; SQ = 1;
                end                
            case 2
                switch m
                    case 1 % |Va| is max
                        S0 = Scc; S1 = Sac; S2 = Sba; SQ = 3;
                    case 2 % |Vb| is max
                        S0 = Scc; S1 = Sab; S2 = Sbc; SQ = 1;
                    otherwise % |Vc| is max
                        S0 = Scc; S1 = Sac; S2 = Sbc; SQ = 2;
                end    
            case 3
                switch m
                    case 1 % |Va| is max
                        S0 = Sbb; S1 = Sac; S2 = Sba; SQ = 1;
                    case 2 % |Vb| is max
                        S0 = Sbb; S1 = Sbc; S2 = Sba; SQ = 2;
                    otherwise % |Vc| is max
                        S0 = Sbb; S1 = Sbc; S2 = Sca; SQ = 3;
                end
            case 4
                switch m
                    case 1 % |Va| is max
                        S0 = Saa; S1 = Sba; S2 = Sca; SQ = 2;
                    case 2 % |Vb| is max
                        S0 = Saa; S1 = Sba; S2 = Scb; SQ = 3;
                    otherwise % |Vc| is max
                        S0 = Saa; S1 = Sbc; S2 = Sca; SQ = 1;
                end
            case 5
                switch m
                    case 1 % |Va| is max
                        S0 = Scc; S1 = Sca; S2 = Sab; SQ = 3;
                    case 2 % |Vb| is max
                        S0 = Scc; S1 = Sba; S2 = Scb; SQ = 1;
                    otherwise % |Vc| is max
                        S0 = Scc; S1 = Sca; S2 = Scb; SQ = 2;
                end
            case 6
                switch m
                    case 1 % |Va| is max
                        S0 = Sbb; S1 = Sca; S2 = Sab; SQ = 1;
                    case 2 % |Vb| is max
                        S0 = Sbb; S1 = Scb; S2 = Sab; SQ = 2;
                    otherwise % |Vc| is max
                        S0 = Sbb; S1 = Scb; S2 = Sac; SQ = 3;
                end               
            otherwise
                S0 = Saa; S1 = Sab; S2 = Sac; SQ = 0;
        end
        
%%        
        % initialize switching functions
        Sap = 1; Sbp = 1; Scp = 1;
        San = 1; Sbn = 1; Scn = 1;

        % Calculate T1 T2 for SQ1 and SQ3
        T1_SQ1 = T1;
        T2_SQ1 = T1 + T2;
        T0_SQ1 = Ts - T1_SQ1 - T2_SQ1;
        
        T1_SQ3 = T1 + T2;
        T2_SQ3 = T2;
        T0_SQ3 = Ts - T1_SQ3 - T2_SQ3;
        
        % Assign TZ TA TB
        switch SQ
            case 1
                TZ = T0_SQ1; TA = T1_SQ1; TB = T2_SQ1;
            case 2
                TZ = T0; TA = T1; TB = T2;
            otherwise
                TZ = T0_SQ3; TA = T1_SQ3; TB = T2_SQ3;                
        end
        
        % PWM sequence: IA-IZ-IB-IZ-IA
            if TT>=0 && TT<TA/2
                % T1
                Sap = S1(1);    Sbp = S1(2);    Scp = S1(3);
                San = S1(4);    Sbn = S1(5);    Scn = S1(6);

            elseif TT>=TA/2 && TT<TA/2 + TZ/2
                % T0
                Sap = S0(1);    Sbp = S0(2);    Scp = S0(3);
                San = S0(4);    Sbn = S0(5);    Scn = S0(6);    

            elseif TT>=TA/2 + TZ/2 && TT<=TA/2 + TZ/2 + TB 
                % T2
                Sap = S2(1);    Sbp = S2(2);    Scp = S2(3);
                San = S2(4);    Sbn = S2(5);    Scn = S2(6);
    
            elseif TT>=TA/2 + TZ/2 + TB && TT<TA/2 + TZ + TB
                % T0 state
                Sap = S0(1);    Sbp = S0(2);    Scp = S0(3);
                San = S0(4);    Sbn = S0(5);    Scn = S0(6);

            elseif TT>=TA/2 + TZ + TB && TT<Ts
                % T1
                Sap = S1(1);    Sbp = S1(2);    Scp = S1(3);
                San = S1(4);    Sbn = S1(5);    Scn = S1(6);
            end        
    end

%% ASVM: 2023 APEC, reduction of CMV and switching losses
% ASVM
    function [Sap, Sbp, Scp, San, Sbn, Scn, Seq] = ASVM(k,TT,Ts,Saa,Sbb,Scc,Sab,Sac,Sbc,Sba,Sca,Scb,Va,Vb,Vc)
        Va_mag = abs(Va);
        Vb_mag = abs(Vb);
        Vc_mag = abs(Vc);
        
        Vab_mag = abs(Va-Vb);
        Vbc_mag = abs(Vb-Vc);
        Vca_mag = abs(Vc-Va);
        
        n = mod(k,3);
        
        % initialize switching functions
        Sap = 1; Sbp = 1; Scp = 1;
        San = 1; Sbn = 1; Scn = 1;
       
        %%% START MIN VOLTAGE IDENFICATION %%%
        % Vmin = |Va|
        if(Vc_mag >= Vb_mag && Vb_mag >= Va_mag) 
            m = 1; % |Va| = |Vb| = |Vc| is considered Vmin = |Va|
        elseif(Vb_mag >= Vc_mag && Vc_mag >= Va_mag)
            m = 1; % |Vb| > |Va| >= |Vc|
            if(Vb_mag > Vc_mag && Vc_mag == Va_mag)
                m = 3;
            end
        % Vmin = |Vb|    
        elseif(Va_mag >= Vc_mag && Vc_mag > Vb_mag)
            m = 2; % |Vb| >= |Va| > |Vc|
        elseif(Vc_mag >= Va_mag && Va_mag > Vb_mag)
            m = 2;
            if(Vc_mag > Va_mag && Va_mag == Vb_mag)
                m = 1;
            end
        % Vmin = |Vc|    
        elseif(Vb_mag >= Va_mag && Va_mag > Vc_mag)
            m = 3;
        elseif(Va_mag >= Vb_mag && Vb_mag > Vc_mag)
            m = 3;
            if(Va_mag > Vb_mag && Vb_mag == Vc_mag)
                m = 2;
            end
        else
            m = 0;
        end
        %%% END MIN VOLTAGE IDENTIFICAION %%%
        
        
        %%% START S0 allocation %%%
        switch m
            case 1 % Vmin = |Va|
                S0 = Saa;
            case 2 % Vmin = |Vb|
                S0 = Sbb;
            otherwise
                S0 = Scc;
        end
        %%% END S0 allocation %%%
        
        %%% SEQUENCE ALLOCATION %%%
        switch n % sector number in mod
            case 1
                if(m == 2)
                    Seq = 1; % CSM1A
                elseif(m ==3)
                    Seq = 2; % CSM1B
                else % m == 1
                    if(Vca_mag>=Vab_mag)
                        Seq = 1;
                    else
                        Seq = 2;
                    end
                end
            case 2
                if(m == 1)
                    Seq = 1; % CSM1A
                elseif(m ==2)
                    Seq = 2; % CSM1B
                else % m == 3
                    if(Vbc_mag>=Vca_mag)
                        Seq = 1;
                    else
                        Seq = 2;
                    end
                end
            otherwise % case 3 where k = 3 or 6
                if(m == 1) % min = |Va|
                    Seq = 2; % CSM1A
                elseif(m == 3) % min = |Vc|
                    Seq = 1; % CSM1B
                else % m == 2 whic is min = |Vb|
                    if(Vab_mag>=Vbc_mag)
                        Seq = 1;
                    else
                        Seq = 2;
                    end
                end
        end
        %%% END SEQUENCE ALLOCATION %%%
      
%%        
        switch k
            case 1
                S1 = Sab; S2 = Sac;
            case 2
                S1 = Sac; S2 = Sbc;
            case 3
                S1 = Sbc; S2 = Sba;
            case 4
                S1 = Sba; S2 = Sca;
            case 5
                S1 = Sca; S2 = Scb;
            case 6
                S1 = Scb; S2 = Sab;
            otherwise
                S1 = Sab; S2 = Sac;
        end        
        
        switch Seq
            case 1 % CSM1A PWM sequence: IZ-IA-IB-IA-IZ
                if TT>=0 && TT<T0/2
                    % aa or bb or cc, CSI zero state
                Sap = S0(1);    Sbp = S0(2);    Scp = S0(3);
                San = S0(4);    Sbn = S0(5);    Scn = S0(6);

            elseif TT>=T0/2 && TT<T0/2 + T1/2
                % T1 state
                Sap = S1(1);    Sbp = S1(2);    Scp = S1(3);
                San = S1(4);    Sbn = S1(5);    Scn = S1(6);    

            elseif TT>=T0/2 + T1/2 && TT<=T0/2 + T1/2 +T2 
                % T2 state
                Sap = S2(1);    Sbp = S2(2);    Scp = S2(3);
                San = S2(4);    Sbn = S2(5);    Scn = S2(6);
    
            elseif TT>=T0/2 + T1/2 +T2 && TT<T0/2 + T1 +T2
                % T1 state
                Sap = S1(1);    Sbp = S1(2);    Scp = S1(3);
                San = S1(4);    Sbn = S1(5);    Scn = S1(6);

            elseif TT>=T0/2 + T1 +T2 && TT<Ts
                % aa or bb or cc, CSI zero state
                Sap = S0(1);    Sbp = S0(2);    Scp = S0(3);
                San = S0(4);    Sbn = S0(5);    Scn = S0(6);
                end
                
            otherwise % CSM1B
                if TT>=0 && TT<T0/2
                    % aa or bb or cc, CSI zero state
                    Sap = S0(1);    Sbp = S0(2);    Scp = S0(3);
                    San = S0(4);    Sbn = S0(5);    Scn = S0(6);

                elseif TT>=T0/2 && TT<T0/2 + T2/2
                    % T1 state
                    Sap = S2(1);    Sbp = S2(2);    Scp = S2(3);
                    San = S2(4);    Sbn = S2(5);    Scn = S2(6);    

                elseif TT>=T0/2 + T2/2 && TT<=T0/2 + T2/2 +T1 
                % T2 state
                Sap = S1(1);    Sbp = S1(2);    Scp = S1(3);
                San = S1(4);    Sbn = S1(5);    Scn = S1(6);
    
                elseif TT>=T0/2 + T2/2 +T1 && TT<T0/2 + T2 +T1
                % T1 state
                Sap = S2(1);    Sbp = S2(2);    Scp = S2(3);
                San = S2(4);    Sbn = S2(5);    Scn = S2(6);

                elseif TT>=T0/2 + T2 + T1 && TT<Ts
                % aa or bb or cc, CSI zero state
                Sap = S0(1);    Sbp = S0(2);    Scp = S0(3);
                San = S0(4);    Sbn = S0(5);    Scn = S0(6);
                end  
        end
    end

end % End of PWM BOX function
